simulink model "lsr_id"  (R2024b)
settings: Solver=VariableStepAuto  StartTime=0.0  StopTime=inf  RelTol=1e-3
undefined symbols (not defined in the file or in its folder): canChannel, dspblkCoreblockFVToolHelper, gcbh
libraries: canmsglib x6, ros2lib x4, canlib x2
settings Model: Creator=gem  LastModifiedBy=gem

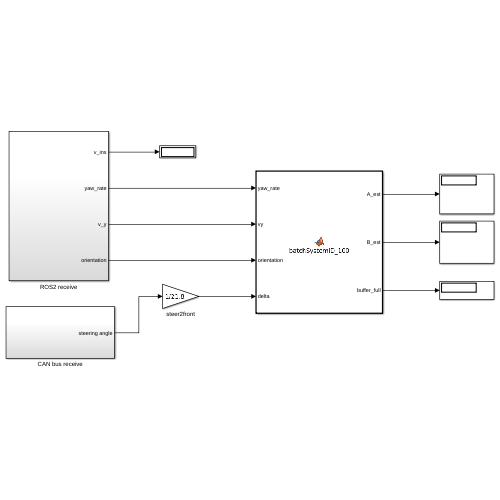
[thumbnail: Simulink's stored preview of the top-level diagram]
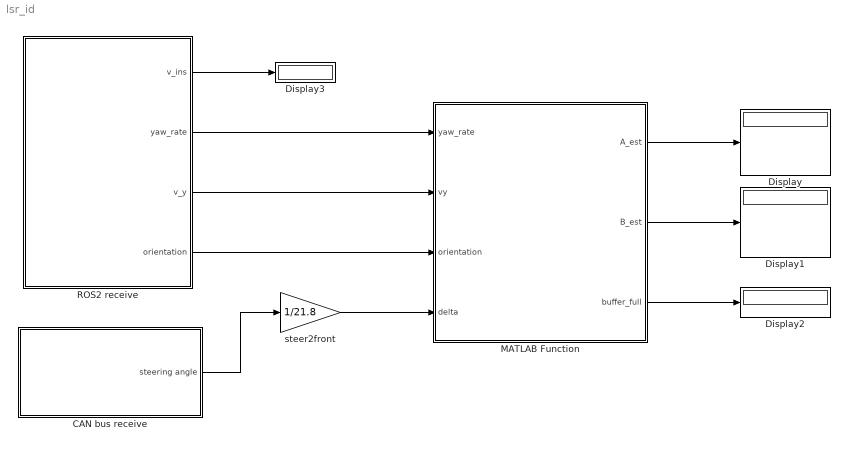
== system lsr_id ==
  CAN bus receive : Subsystem
  Display{,1..3} (4 alike) : Display
  MATLAB Function : MATLAB Function  TreatAsAtomicUnit=on
  ROS2 receive : Subsystem
  steer2front : Gain  Gain=1/21.8  OutDataTypeStr=single
  wires:
  ROS2 receive/3(v_y) -> MATLAB Function/2(vy)
  ROS2 receive/2(yaw_rate) -> MATLAB Function/1(yaw_rate)
  MATLAB Function/1(A_est) -> Display/1
  MATLAB Function/2(B_est) -> Display1/1
  MATLAB Function/3(buffer_full) -> Display2/1
  CAN bus receive/1(steering angle) -> steer2front/1
  ROS2 receive/1(v_ins) -> Display3/1
  steer2front/1 -> MATLAB Function/4(delta)
  ROS2 receive/4(orientation) -> MATLAB Function/3(orientation)

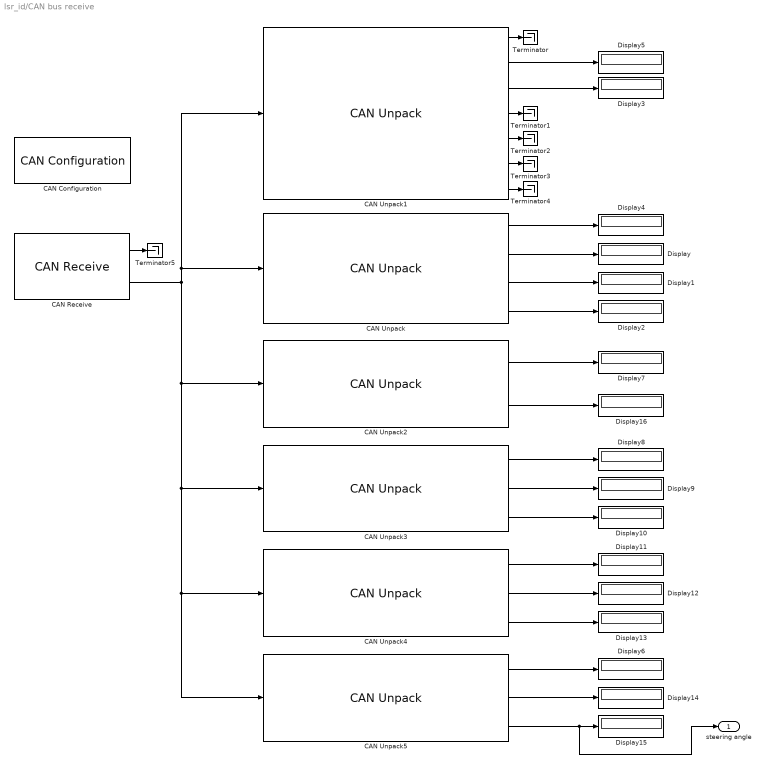
== system lsr_id/CAN bus receive ==
  CAN Configuration : canlib/CAN Configuration  BlockHandle=156.0001  Device=MathWorks Virtual 1 (Channel 1)  DeviceMenu=MathWorks Virtual 1 (Channel 1)  ObjConstructor=canChannel('MathWorks', 'Virtual 1', 1)  BusSpeed=500000  EnableBitParameters=off  AckMode=Normal
  CAN Receive : canlib/CAN Receive  BlockHandle=157.0001  Device=MathWorks Virtual 1 (Channel 1)  DeviceMenu=MathWorks Virtual 1 (Channel 1)  ObjConstructor=canChannel('MathWorks', 'Virtual 1', 1)  EnableStandardIDsFilter=off  StdIDsCombo=Allow all  StandardIDs=0  EnableExtendedIDsFilter=off  ExtIDsCombo=Allow all  ExtendedIDs=0  SampleTime=0.01  MsgsPerTimestep=all  InternalFilterUpdateStatus=on  BusOutput=off
  CAN Unpack : canmsglib/CAN Unpack  CANdbFile=/home/gem/Gem_Simulink_ws/utilities/as_pacmod_v2.dbc  MsgList=BRAKE_RPT  MsgName=BRAKE_RPT  MsgIDType=Standard (11-bit identifier)  MsgIdentifier=108  MsgLength=8  SignalInfo={'BRAKE_ON_OFF','48','1','BE','unsigned','Standard','0','1','0','0','1';'COMMANDED_VALUE','24','16','BE','unsigned','Standard','0','0.001','0','0','1';'MANUAL_INPUT','8','16','BE','unsigned','Standard','0','0.001','0','0','1';'OUTPUT_VALUE','40','16','BE','unsigned','Standard','0','0.001','0','0','1'}  IDPort=off  TimestampPort=off  ErrorPort=off  RemotePort=off  LengthPort=off  StatusPort=off  ApplyMinMax=off
      settings: DataFormat=CANdb specified signals
  CAN Unpack1 : canmsglib/CAN Unpack  CANdbFile=/home/gem/Gem_Simulink_ws/utilities/as_pacmod_v2.dbc  MsgList=GLOBAL_RPT  MsgName=GLOBAL_RPT  MsgIDType=Standard (11-bit identifier)  MsgIdentifier=106  MsgLength=8  SignalInfo={'BRK_CAN_TIMEOUT','4','1','BE','unsigned','Standard','0','1','0','0','1';'OVERRIDE_STATUS','1','1','BE','unsigned','Standard','0','1','0','0','1';'PACMOD_STATUS','0','1','BE','unsigned','Standard','0','1','0','0','1';'STR_CAN_TIMEOUT','3','1','BE','unsigned','Standard','0','1','0','0','1';'USR_CAN_READ_ERRORS','56','16','BE','unsigned','Standard','0','1','0','0','65535';'USR_CAN_TIMEOUT','5','1','BE','unsigned','Standard','0','1','0','0','1';'VEH_CAN_TIMEOUT','2','1','BE','unsigned','Standard','0','1','0','0','1'}  IDPort=off  TimestampPort=off  ErrorPort=off  RemotePort=off  LengthPort=off  StatusPort=off  ApplyMinMax=off
      settings: DataFormat=CANdb specified signals
  CAN Unpack2 : canmsglib/CAN Unpack  CANdbFile=/home/gem/Gem_Simulink_ws/utilities/as_pacmod_v2.dbc  MsgList=VEHICLE_SPEED_RPT  MsgName=VEHICLE_SPEED_RPT  MsgIDType=Standard (11-bit identifier)  MsgIdentifier=111  MsgLength=8  SignalInfo={'VEHICLE_SPEED','8','16','BE','signed','Standard','0','0.01','0','-327.68','327.67';'VEHICLE_SPEED_VALID','16','1','BE','unsigned','Standard','0','1','0','0','1'}  IDPort=off  TimestampPort=off  ErrorPort=off  RemotePort=off  LengthPort=off  StatusPort=off  ApplyMinMax=off
      settings: DataFormat=CANdb specified signals
  CAN Unpack3 : canmsglib/CAN Unpack  CANdbFile=/home/gem/Gem_Simulink_ws/utilities/as_pacmod_v2.dbc  MsgList=ACCEL_RPT  MsgName=ACCEL_RPT  MsgIDType=Standard (11-bit identifier)  MsgIdentifier=104  MsgLength=8  SignalInfo={'COMMANDED_VALUE','24','16','BE','unsigned','Standard','0','0.001','0','0','1';'MANUAL_INPUT','8','16','BE','unsigned','Standard','0','0.001','0','0','1';'OUTPUT_VALUE','40','16','BE','unsigned','Standard','0','0.001','0','0','1'}  IDPort=off  TimestampPort=off  ErrorPort=off  RemotePort=off  LengthPort=off  StatusPort=off  ApplyMinMax=off
      settings: DataFormat=CANdb specified signals
  CAN Unpack4 : canmsglib/CAN Unpack  CANdbFile=/home/gem/Gem_Simulink_ws/utilities/as_pacmod_v2.dbc  MsgList=SHIFT_RPT  MsgName=SHIFT_RPT  MsgIDType=Standard (11-bit identifier)  MsgIdentifier=102  MsgLength=8  SignalInfo={'COMMANDED_VALUE','8','8','BE','unsigned','Standard','0','1','0','0','4';'MANUAL_INPUT','0','8','BE','unsigned','Standard','0','1','0','0','4';'OUTPUT_VALUE','16','8','BE','unsigned','Standard','0','1','0','0','4'}  IDPort=off  TimestampPort=off  ErrorPort=off  RemotePort=off  LengthPort=off  StatusPort=off  ApplyMinMax=off
      settings: DataFormat=CANdb specified signals
  CAN Unpack5 : canmsglib/CAN Unpack  CANdbFile=/home/gem/Gem_Simulink_ws/utilities/as_pacmod_v2.dbc  MsgList=STEERING_RPT_1  MsgName=STEERING_RPT_1  MsgIDType=Standard (11-bit identifier)  MsgIdentifier=110  MsgLength=8  SignalInfo={'COMMANDED_VALUE','24','16','BE','signed','Standard','0','0.001','0','-32.768','32.767';'MANUAL_INPUT','8','16','BE','signed','Standard','0','0.001','0','-32.768','32.767';'OUTPUT_VALUE','40','16','BE','signed','Standard','0','0.001','0','-32.768','32.767'}  IDPort=off  TimestampPort=off  ErrorPort=off  RemotePort=off  LengthPort=off  StatusPort=off  ApplyMinMax=off
      settings: DataFormat=CANdb specified signals
  Display{,1..16} (17 alike) : Display
  Terminator{,1..5} (6 alike) : Terminator
  steering angle : Outport
  wires:
  CAN Unpack/3 -> Display1/1
  CAN Unpack1/2 -> Display5/1
  CAN Unpack3/2 -> Display9/1
  CAN Unpack1/4 -> Terminator1/1
  CAN Unpack/4 -> Display2/1
  CAN Unpack2/1 -> Display7/1
  CAN Unpack1/7 -> Terminator4/1
  CAN Unpack5/3 -> steering angle/1, Display15/1
  CAN Unpack2/2 -> Display16/1
  CAN Unpack/2 -> Display/1
  CAN Unpack1/6 -> Terminator3/1
  CAN Unpack3/3 -> Display10/1
  CAN Unpack5/1 -> Display6/1
  CAN Unpack4/2 -> Display12/1
  CAN Unpack1/1 -> Terminator/1
  CAN Receive/1 -> Terminator5/1
  CAN Unpack/1 -> Display4/1
  CAN Unpack1/3 -> Display3/1
  CAN Receive/2 -> CAN Unpack1/1, CAN Unpack/1, CAN Unpack5/1, CAN Unpack4/1, CAN Unpack3/1, CAN Unpack2/1
  CAN Unpack4/1 -> Display11/1
  CAN Unpack1/5 -> Terminator2/1
  CAN Unpack3/1 -> Display8/1
  CAN Unpack5/2 -> Display14/1
  CAN Unpack4/3 -> Display13/1

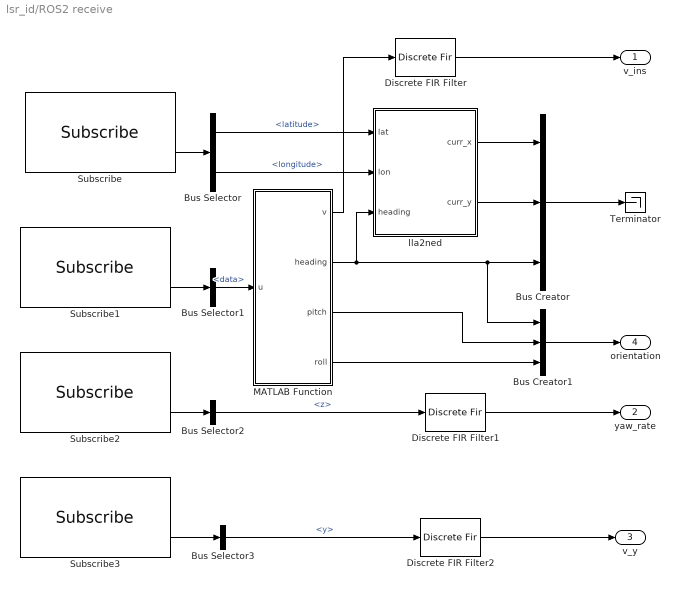
== system lsr_id/ROS2 receive ==
  Bus Creator : BusCreator  Inputs=3
  Bus Creator1 : BusCreator  Inputs=3
  Bus Selector : BusSelector  OutputSignals=latitude,longitude
  Bus Selector1 : BusSelector  OutputSignals=data
  Bus Selector2 : BusSelector  OutputSignals=angular_velocity.z
  Bus Selector3 : BusSelector  OutputSignals=twist.twist.linear.y
  Discrete FIR Filter : DiscreteFir  LoadFcn=dspblkCoreblockFVToolHelper(gcbh,'load');  Coefficients=[0.5 0.3 0.2]
      settings: CopyFcn=dspblkCoreblockFVToolHelper(gcbh,'copy');  DeleteFcn=dspblkCoreblockFVToolHelper(gcbh,'close');  ModelCloseFcn=dspblkCoreblockFVToolHelper(gcbh,'close');  PreSaveFcn=dspblkCoreblockFVToolHelper(gcbh,'presave');  PostSaveFcn=dspblkCoreblockFVToolHelper(gcbh,'postsave');  CloseFcn=dspblkCoreblockFVToolHelper(gcbh,'close');
  Discrete FIR Filter1 : DiscreteFir  LoadFcn=dspblkCoreblockFVToolHelper(gcbh,'load');  Coefficients=[0.5 0.3 0.2]
      settings: CopyFcn=dspblkCoreblockFVToolHelper(gcbh,'copy');  DeleteFcn=dspblkCoreblockFVToolHelper(gcbh,'close');  ModelCloseFcn=dspblkCoreblockFVToolHelper(gcbh,'close');  PreSaveFcn=dspblkCoreblockFVToolHelper(gcbh,'presave');  PostSaveFcn=dspblkCoreblockFVToolHelper(gcbh,'postsave');  CloseFcn=dspblkCoreblockFVToolHelper(gcbh,'close');
  Discrete FIR Filter2 : DiscreteFir  LoadFcn=dspblkCoreblockFVToolHelper(gcbh,'load');  Coefficients=[0.5 0.3 0.2]
      settings: CopyFcn=dspblkCoreblockFVToolHelper(gcbh,'copy');  DeleteFcn=dspblkCoreblockFVToolHelper(gcbh,'close');  ModelCloseFcn=dspblkCoreblockFVToolHelper(gcbh,'close');  PreSaveFcn=dspblkCoreblockFVToolHelper(gcbh,'presave');  PostSaveFcn=dspblkCoreblockFVToolHelper(gcbh,'postsave');  CloseFcn=dspblkCoreblockFVToolHelper(gcbh,'close');
  MATLAB Function : MATLAB Function  TreatAsAtomicUnit=on
  Subscribe : ros2lib/Subscribe  topicSource=Select from ROS network  topic=/navsatfix  messageType=sensor_msgs/NavSatFix  sampleTime=-1  QOSHistory=Keep last  QOSDepth=1  QOSReliability=Reliable  QOSDurability=Volatile  QOSDeadline=Inf  QOSLifespan=Inf  QOSLiveliness=Automatic  QOSLeaseDuration=Inf  QOSAvoidROSNamespaceConventions=off
  Subscribe1 : ros2lib/Subscribe  topicSource=Select from ROS network  topic=/ins_info  messageType=std_msgs/Float64MultiArray  sampleTime=-1  QOSHistory=Keep last  QOSDepth=1  QOSReliability=Reliable  QOSDurability=Volatile  QOSDeadline=Inf  QOSLifespan=Inf  QOSLiveliness=Automatic  QOSLeaseDuration=Inf  QOSAvoidROSNamespaceConventions=off
  Subscribe2 : ros2lib/Subscribe  topicSource=Select from ROS network  topic=/imu  messageType=sensor_msgs/Imu  sampleTime=-1  QOSHistory=Keep last  QOSDepth=1  QOSReliability=Reliable  QOSDurability=Volatile  QOSDeadline=Inf  QOSLifespan=Inf  QOSLiveliness=Automatic  QOSLeaseDuration=Inf  QOSAvoidROSNamespaceConventions=off
  Subscribe3 : ros2lib/Subscribe  topicSource=Select from ROS network  topic=/localization  messageType=nav_msgs/Odometry  sampleTime=-1  QOSHistory=Keep last  QOSDepth=1  QOSReliability=Reliable  QOSDurability=Volatile  QOSDeadline=Inf  QOSLifespan=Inf  QOSLiveliness=Automatic  QOSLeaseDuration=Inf  QOSAvoidROSNamespaceConventions=off
  Terminator : Terminator
  lla2ned : MATLAB Function  TreatAsAtomicUnit=on
  v_ins : Outport
  yaw_rate : Outport  Port=2
  v_y : Outport  Port=3
  orientation : Outport  Port=4
  wires:
  lla2ned/2(curr_y) -> Bus Creator/2
  lla2ned/1(curr_x) -> Bus Creator/1
  Subscribe/2 -> Bus Selector/1
  Bus Selector/1 -> lla2ned/1(lat)  "<latitude>"
  Bus Selector/2 -> lla2ned/2(lon)  "<longitude>"
  Subscribe1/2 -> Bus Selector1/1
  Bus Selector1/1 -> MATLAB Function/1(u)  "<data>"
  MATLAB Function/2(heading) -> lla2ned/3(heading), Bus Creator1/1, Bus Creator/3
  MATLAB Function/1(v) -> Discrete FIR Filter/1
  Discrete FIR Filter/1 -> v_ins/1
  Subscribe2/2 -> Bus Selector2/1
  Bus Selector2/1 -> Discrete FIR Filter1/1  "<z>"
  Discrete FIR Filter1/1 -> yaw_rate/1
  Bus Creator/1 -> Terminator/1
  Subscribe3/2 -> Bus Selector3/1
  Bus Selector3/1 -> Discrete FIR Filter2/1  "<y>"
  Discrete FIR Filter2/1 -> v_y/1
  MATLAB Function/3(pitch) -> Bus Creator1/2
  MATLAB Function/4(roll) -> Bus Creator1/3
  Bus Creator1/1 -> orientation/1

== matlab function lsr_id/ROS2 receive/lla2ned ==
  data: curr_x output; lat input; curr_y output; lon input; heading input
function [curr_x, curr_y]= fcn(lat, lon, heading)

lat0 = 40.0928149;
lon0 = -88.235940;
alt0 = 203.0;
offset = 2.56;

lla0 = [lat0 lon0 alt0];
lla = [lat, lon, alt0];

xyzNED = lla2ned(lla,lla0,'flat');

if heading >= 270 && heading < 360
    yaw_curr = deg2rad(450 - heading);
else
    yaw_curr = deg2rad(90 - heading);
end

curr_x = xyzNED(2) + offset*cos(yaw_curr);
curr_y = xyzNED(1) + offset*sin(yaw_curr);

== matlab function lsr_id/MATLAB Function ==
  data: yaw_rate input; vy input; orientation input; delta input; A_est output; B_est output; buffer_full output
function [A_est, B_est, buffer_full] = batchSystemID_100(yaw_rate, vy, orientation, delta)
    % Inputs:
    % pitch, roll      - Current pitch and roll angles
    % vy, yaw_rate     - Current lateral speed and yaw rate
    % delta            - Current steering angle
    % reset            - Signal to reset the buffer and reinitialize

    % Outputs:
    % A_est, B_est     - Estimated state-space matrices A and B
    % buffer_full      - Flag indicating if the buffer is full and identification is performed

    % Persistent variables for buffering data and storing previous estimates
    persistent x_prev_buffer u_buffer x_curr_buffer pitch_buffer roll_buffer ...
               data_count A_est_prev B_est_prev

    pitch = orientation(2);
    roll = orientation(3);

    if isempty(x_prev_buffer)
        % Initialize buffers and counters
        x_prev_buffer = zeros(2, 100); % Buffer for previous states [vy_prev; yaw_rate_prev]
        u_buffer = zeros(1, 100);      % Buffer for steering angle (control input)
        x_curr_buffer = zeros(2, 100); % Buffer for current states [vy; yaw_rate]
        pitch_buffer = zeros(1, 100);  % Buffer for pitch angle
        roll_buffer = zeros(1, 100);   % Buffer for roll angle
        data_count = 0;                % Counter for data points collected
        A_est_prev = zeros(2, 2);      % Previous A matrix estimate
        B_est_prev = zeros(2, 1);      % Previous B matrix estimate
    end

    % Update the buffer
    if data_count < 100
        data_count = data_count + 1;
        x_prev_buffer(:, data_count) = [vy; yaw_rate];
        u_buffer(:, data_count) = delta;
        pitch_buffer(:, data_count) = pitch;
        roll_buffer(:, data_count) = roll;
        if data_count > 1
            x_curr_buffer(:, data_count - 1) = [vy; yaw_rate];
        end
    end

    % Check if buffer is full
    buffer_full = (data_count == 100);
    if buffer_full
        % Validate pitch and roll stability
        if std(pitch_buffer) < 0.4 && std(roll_buffer) < 0.4
            % Prepare regression matrices
            Phi = [x_prev_buffer(:, 1:99); u_buffer(:, 1:99)]'; % Regressor matrix
            Y = x_curr_buffer(:, 1:99)';                       % Output matrix

            % Solve for theta using least squares
            theta = (Phi' * Phi) \ (Phi' * Y); % Regression coefficients

            % Extract A and B matrices
            A_est = theta(1:2, :)'; % A: First two columns
            B_est = theta(3, :)';   % B: Last column

            % Update previous estimates
            A_est_prev = A_est;
            B_est_prev = B_est;
        else
            % Invalid data: Clear buffers and reset data count
            x_prev_buffer = zeros(2, 100);
            u_buffer = zeros(1, 100);
            x_curr_buffer = zeros(2, 100);
            pitch_buffer = zeros(1, 100);
            roll_buffer = zeros(1, 100);
            data_count = 0;

            % Output previous estimates
            A_est = A_est_prev;
            B_est = B_est_prev;
        end

        % Reset data count after identification or invalidation
        data_count = 0;
    else
        % Output previous estimates if buffer is not full
        A_est = A_est_prev;
        B_est = B_est_prev;
    end
end

== matlab function lsr_id/ROS2 receive/MATLAB Function ==
  data: v output; u input; heading output; pitch output; roll output
function [v, heading, pitch, roll] = fcn(u)
v = u(1);
heading = u(2);
pitch = u(3);
roll = u(4);
